simulink model "real_time_simulink_Part34"  (R2024b)
settings: Solver=ode5  StartTime=0.0  StopTime=1  FixedStep=0.001  RelTol=1e-3
InitFcn:
  | Design34
values from neighbouring files (symbols this model uses):
  Cprime = [1, 0, 0, 0]    [Design12.m]    (also in Design34.m)
  K = [58.28, 17.91, 2.58, 1.04]    [Design12.m]    (also in Design34.m = TmpK(2:end))
  Ki = TmpK(1)    [Design34.m]
  Nr = Nu + K * Nx    [Design12.m]    (also in Design34.m)
  t0 = 0.2    [Design12.m]    (also in Design34.m)
  t1 = 0.7    [Design12.m]    (also in Design34.m)
undefined symbols (not defined in the file or in its folder): DiscIntNeverNeededParam, Estimator, National_Instruments, PCI, pulse2deg
libraries: simulink_extras x5, sldrtlib x3, simulink x1
settings Model: SimulationMode=external  ExtModeTrigDuration=1000001  Creator=galeazzolu  LastModifiedBy=galeazzolu
settings DataIOCC: ReturnWorkspaceOutputs=off
settings HardwareCC: ProdBitPerLong=64  ProdHWDeviceType=Intel->x86-64 (Linux 64)
settings RTWCC: Description=Simulink Desktop Real-Time  SystemTargetFile=sldrt.tlc  TemplateMakefile=sldrt.tmf  RTWCompilerOptimization=on
settings CodeAppCC: MaxIdLength=95
settings SimulinkDesktopRealTimeCC: TargetLibSuffix=_sldrt.a  TargetPreCompLibLocation=C:\Program Files\MATLAB\R2024b\toolbox\sldrt\lib\win64  ParMdlRefBuildCompliant=on

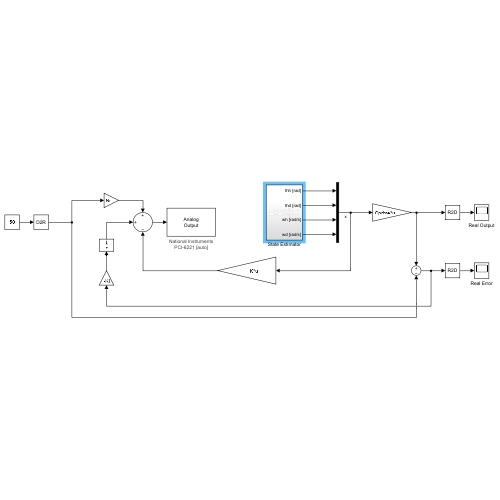
[thumbnail: Simulink's stored preview of the top-level diagram]
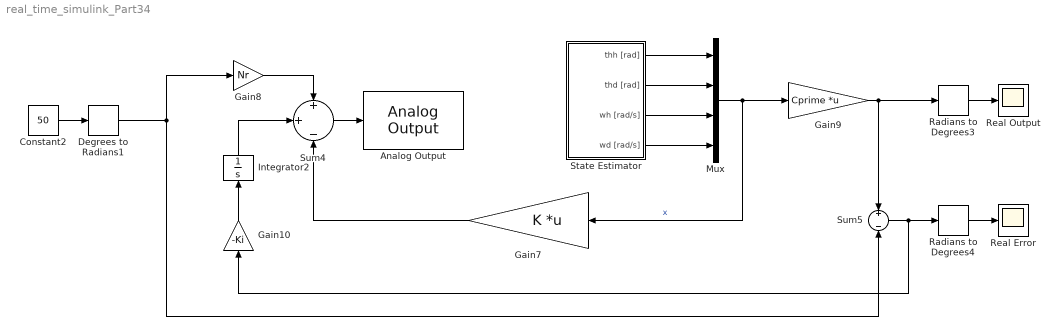
== system real_time_simulink_Part34 ==
  Analog Output : sldrtlib/Analog Output  SampleTime=-1  MaxMissedTicks=10  ShowMissedTicks=off  YieldWhenWaiting=off  DrvName=National_Instruments/PCI-6221  DrvAddress=4294967295  DrvOptions=[0 0 0 2 0]  Channels=1  RangeMode=1  VoltRange=1  InitialValue=0  FinalValue=0
      settings: AttributesFormatString=National Instruments\nPCI-6221 [auto]
  Constant2 : Constant  Value=50
  Degrees to Radians1 : simulink_extras/Transformations/Degrees to Radians
  Gain10 : Gain  Gain=-Ki
  Gain7 : Gain  Gain=K  Multiplication=Matrix(K*u)
  Gain8 : Gain  Gain=Nr
  Gain9 : Gain  Gain=Cprime  Multiplication=Matrix(K*u)
  Integrator2 : Integrator
  Mux : Mux
  Radians to Degrees3 : simulink_extras/Transformations/Radians to Degrees
  Radians to Degrees4 : simulink_extras/Transformations/Radians to Degrees
  Real Error : Scope
  Real Output : Scope
  State Estimator : Subsystem
  Sum4 : Sum  Inputs=+|+|-
  Sum5 : Sum  Inputs=+||-
  wires:
  State Estimator/3(wh [rad/s]) -> Mux/3
  Gain10/1 -> Integrator2/1
  Radians to Degrees4/1 -> Real Error/1
  Radians to Degrees3/1 -> Real Output/1
  State Estimator/2(thd [rad]) -> Mux/2
  Constant2/1 -> Degrees to Radians1/1
  Gain8/1 -> Sum4/1
  Degrees to Radians1/1 -> Sum5/2, Gain8/1
  State Estimator/1(thh [rad]) -> Mux/1
  Integrator2/1 -> Sum4/2
  Sum4/1 -> Analog Output/1
  State Estimator/4(wd [rad/s]) -> Mux/4
  Gain9/1 -> Radians to Degrees3/1, Sum5/1
  Mux/1 -> Gain9/1, Gain7/1  "x"
  Sum5/1 -> Gain10/1, Radians to Degrees4/1
  Gain7/1 -> Sum4/3

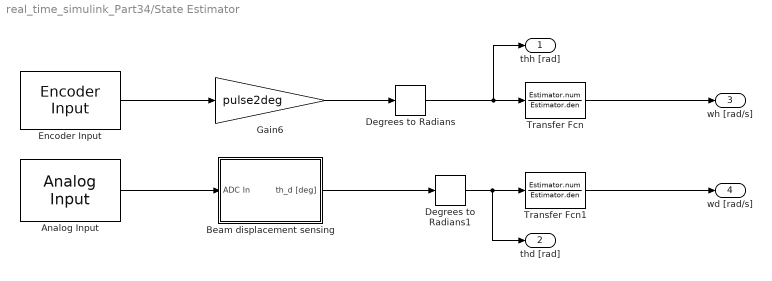
== system real_time_simulink_Part34/State Estimator ==
  Analog Input : sldrtlib/Analog Input  SampleTime=-1  MaxMissedTicks=10  ShowMissedTicks=off  YieldWhenWaiting=off  DrvName=National_Instruments/PCI-6221  DrvAddress=4294967295  DrvOptions=[0 0 0 2 0]  Channels=[3, 4]  RangeMode=1  VoltRange=2  DataType=1
      settings: AttributesFormatString=National Instruments\nPCI-6221 [auto]
  Beam displacement sensing : Subsystem
  Degrees to Radians : simulink_extras/Transformations/Degrees to Radians
  Degrees to Radians1 : simulink_extras/Transformations/Degrees to Radians
  Encoder Input : sldrtlib/Encoder Input  SampleTime=-1  MaxMissedTicks=10  ShowMissedTicks=off  YieldWhenWaiting=off  DrvName=National_Instruments/PCI-6221  DrvAddress=4294967295  DrvOptions=[0 0 0 2 0]  Channels=1  QuadMode=3  IndexPulse=1  InputFilter=Inf  DataType=1
      settings: AttributesFormatString=National Instruments\nPCI-6221 [auto]
  Gain6 : Gain  Gain=pulse2deg
  Transfer Fcn : TransferFcn  Numerator=Estimator.num  Denominator=Estimator.den
  Transfer Fcn1 : TransferFcn  Numerator=Estimator.num  Denominator=Estimator.den
  thh [rad] : Outport
  thd [rad] : Outport  Port=2
  wh [rad/s] : Outport  Port=3
  wd [rad/s] : Outport  Port=4
  wires:
  Transfer Fcn1/1 -> wd [rad/s]/1
  Beam displacement sensing/1(th_d [deg]) -> Degrees to Radians1/1
  Gain6/1 -> Degrees to Radians/1
  Transfer Fcn/1 -> wh [rad/s]/1
  Encoder Input/1 -> Gain6/1
  Degrees to Radians/1 -> thh [rad]/1, Transfer Fcn/1
  Degrees to Radians1/1 -> thd [rad]/1, Transfer Fcn1/1
  Analog Input/1 -> Beam displacement sensing/1(ADC In)

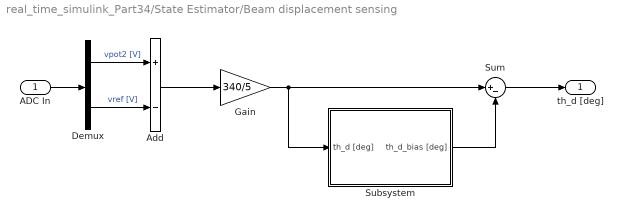
== system real_time_simulink_Part34/State Estimator/Beam displacement sensing ==
  ADC In : Inport
  Add : Sum  Inputs=+-
  Demux : Demux  Outputs=2
  Gain : Gain  Gain=340/5
  Subsystem : Subsystem
  Sum : Sum  Inputs=|+-
  th_d [deg] : Outport
  wires:
  ADC In/1 -> Demux/1
  Demux/1 -> Add/1  "vpot2 [V]"
  Demux/2 -> Add/2  "vref [V]"
  Add/1 -> Gain/1
  Gain/1 -> Subsystem/1(th_d [deg]), Sum/1
  Sum/1 -> th_d [deg]/1
  Subsystem/1(th_d_bias [deg]) -> Sum/2

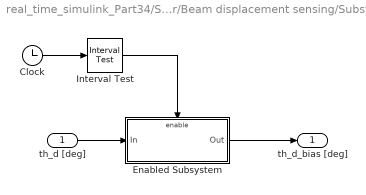
== system real_time_simulink_Part34/State Estimator/Beam displacement sensing/Subsystem ==
  th_d [deg] : Inport
  Clock : Clock
  Enabled Subsystem : Subsystem  TreatAsAtomicUnit=on
  Interval Test : simulink/Logic and Bit Operations/Interval Test  IntervalClosedRight=on  uplimit=t1  IntervalClosedLeft=on  lowlimit=t0  OutDataTypeStr=boolean
  th_d_bias [deg] : Outport
  wires:
  Interval Test/1 -> Enabled Subsystem/Enable
  Clock/1 -> Interval Test/1
  th_d [deg]/1 -> Enabled Subsystem/1(In)
  Enabled Subsystem/1(Out) -> th_d_bias [deg]/1

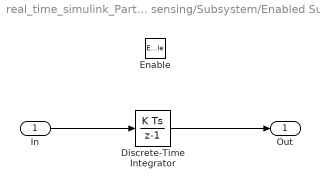
== system real_time_simulink_Part34/State Estimator/Beam displacement sensing/Subsystem/Enabled Subsystem ==
  In : Inport
  Enable : EnablePort
  Discrete-Time Integrator : DiscreteIntegrator  gainval=1/(t1-t0)  SampleTime=-1  ICPrevOutput=DiscIntNeverNeededParam  ICPrevScaledInput=DiscIntNeverNeededParam
  Out : Outport
  wires:
  In/1 -> Discrete-Time Integrator/1
  Discrete-Time Integrator/1 -> Out/1
